simulink model "mm"  (R2023b)
settings: Solver=VariableStepAuto  StartTime=0.0  StopTime=10.0  RelTol=1e-3
undefined symbols (not defined in the file or in its folder): S, vsva2197, xcvc1902
libraries: aieBasic x3, vmcUtilities x1
settings Model: Creator=a.gnaneswaran  LastModifiedBy=a.gnaneswaran

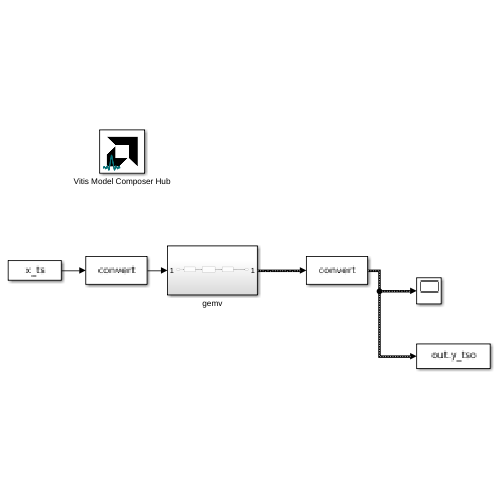
[thumbnail: Simulink's stored preview of the top-level diagram]
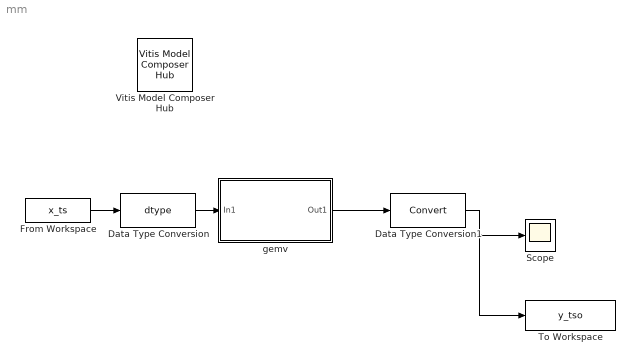
== system mm ==
  Data Type Conversion : DataTypeConversion  OutDataTypeStr=dtype  SaturateOnIntegerOverflow=off  RndMeth=Floor
  Data Type Conversion1 : DataTypeConversion  SaturateOnIntegerOverflow=off  RndMeth=Floor
  From Workspace : FromWorkspace  VariableName=x_ts  OutDataTypeStr=double  SampleTime=1
  Scope : Scope
  To Workspace : ToWorkspace  VariableName=y_tso  SaveFormat=Timeseries  SampleTime=1
      settings: Save2DSignal=2-D array (concatenate along first dimension)
  Vitis Model Composer Hub : vmcUtilities/Vitis Model Composer Hub  Tag=genX  CodeGeneration=off  SubsystemName=gemv  CompilationType=AIECompilation  ExportTypeV2=Graph Code  TargetDirectory=./code  exportDesign=off  analyzeDesign=on  validateDesignOnHw=off  ExportType=AI Engines  IpVendor=xilinx.com  IpLibrary=hls  IpVersion=1.0  IpHWLanguage=Verilog  AieCompilerOptions={}  AieSimulatorOptions={}  CreateTestbench=on  TestbenchStackSize=10  RunRtlSim=off  RunCSim=off  RunAieSim=on  AieSimTimeout=50000  RunAieSimProfiling=off  LaunchVitisAnalyzer=on  PlotOutput=off  RunX86Sim=off  X86SimTimeout=10  GenHwImage=off  GenLibadfXo=off  GenHwValidationCode=off  PlatformType=Not Specified  HwSystemType=Baremetal  HwValidationTarget=hw  ProjDevice=Versal VCK190 Evaluation Platform (xcvc1902-vsva2197-2MP-e-S)  ProjDevicePart=xcvc1902-vsva2197-2MP-e-S  AIEType=AIE  SamplePeriod=-1  ClockFrequency=200  DataPathParallelism=1  xilinxfamily=versalaicore  part=xcvc1902  speed=-2MP-e-S  package=vsva2197  directory=./netlist  testbench=off  incr_netlist=off  synthesis_tool=Vivado  clock_wrapper=Clock Enables  dbl_ovrd=According to Block Masks  dcm_input_clock_period=10  sysclk_period=10  simulink_period=1  eval_field=0  IPInfoJsonString="{\"AIESubsystem\":{\"SubsystemName\":\"gemv\",\"TargetDirectory\":\"./code\",\"SubsystemDir\":\"./code/ip/gemv\"},\"SubsystemTag\":\"AIENode\"}"  LogFileName=/home/a.gnaneswaran/aie_mc/mm/code/model_composer.log  NThreads=4
  gemv : Subsystem
  wires:
  From Workspace/1 -> Data Type Conversion/1
  Data Type Conversion1/1 -> To Workspace/1, Scope/1
  Data Type Conversion/1 -> gemv/1(In1)
  gemv/1(Out1) -> Data Type Conversion1/1

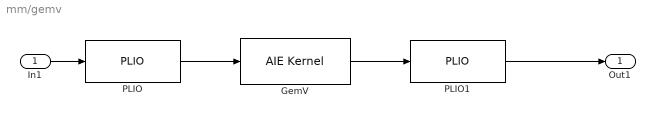
== system mm/gemv ==
  In1 : Inport
  GemV : aieBasic/AIE Kernel  KernelAllAttrs=|  PortNames={'in'; 'out'}  PortSerializedTypes={'{Q2{P{Tinput_stream{1{t{Bi8}}}}}}'; '{Q2{P{Toutput_stream{1{t{Bi8}}}}}}'}  PortWindowSizes={0.000000000000000000e+00, 0.000000000000000000e+00}  PortWindowMargins={0.000000000000000000e+00, 0.000000000000000000e+00}  PortSynchronicities={'auto', 'auto'}  PortSignalSizes={0.000000000000000000e+00; 1.280000000000000000e+02}  FunctionTemplateSpecKind=implicit  FunctionTemplateParamNames={'DX'; 'DY'}  FunctionTemplateParamKinds={'nontype'; 'nontype'}  FunctionTemplateParamTypes={'int'; 'int'}  FunctionTemplateParamValues={'128', '128'}  FunctionIndex=1  FunctionTabVisible=on  FunctionTemplateParamsVisible=on  FunctionDeclTypeOptions=|  FunctionDecl=|  FunctionTemplateParams={ 'DX', 'int', 'DX'; 'DY', 'int', 'DY' }  FunctionTemplateParamsEnables={'off', 'off', 'on';'off', 'off', 'on'}  PortAttrs={ 'input', 'in', 'input_stream_int8 * restrict', '', '', '', ''; 'output', 'out', 'output_stream_int8 * restrict', '', '', '', 'DY' }  PortAttrsEnables={'off', 'off', 'off', 'off', 'off', 'off', 'off';'off', 'off', 'off', 'off', 'off', 'off', 'on'}  SampleTime=-1  KernelHeaderFile=GemV.h  KernelFunction=GemV  KernelSourceFile=GemV.cpp  KernelSearchPaths={}  PreProcOptions={}  blockJsonConstraints="{\"type\":\"constraint\",\"constraintType\":\"stackSize\",\"sid\":\"16\",\"lhs\":{\"type\":\"stackSize\",\"args\":{\"type\":\"kernel\",\"name\":\"mm/gemv/GemV\",\"sid\":\"16\"}},\"rhs\":{\"type\":\"value\",\"args\":{\"type\":\"evaluable\",\"expr\":\"2048\",\"value\":2048}},\"equality\":true}"
      KernelAllAttrs=|
      | s[12;12;9;9;19;14;21;23;21;23;24;21;15;17;12;24;26;26;26;27;28;9;21;23;23;23;24;25;14;19;19;29]@FunctionNameDeclFileNamePortNamesPortTypesPortSerializedTypesPortDirectionsPortWindowSizeEnablesPortWindowMarginEnablesPortBufferSizeEnablesPortBufferMarginEnablesPortSynchronicityEnablesPortSignalSizeEnablesPortBufferSizesPortBufferMarginsFunctionDeclFunctionTemplateSpecKindFunctionTemplateParamNamesFunctionTemplateParamKindsFunctionTemplateParamTypesFunctionTemplateParamValuesFunctionTemplateParamEnablesClassDeclClassTemplateSpecKindClassTemplateParamNamesClassTemplateParamKindsClassTemplateParamTypesClassTemplateParamValuesClassTemplateParamEnablesClassCtorDeclsClassCtorParamNamesClassCtorParamTypesClassCtorParamSerializedTypes[1 1]@C[32 1]@t4@GemVt12@../../GemV.hC[2 1]@t2@int3@outC[2 1]@t28@input_stream_int8 * restrictt29@output_stream_int8 * restrictC[2 1]@t33@{Q2{P{Tinput_stream{1{t{Bi8}}}}}}t34@{Q2{P{Toutput_stream{1{t{Bi8}}}}}}C[2 1]@t5@inputt6@outputC[2 1]@l0@l0@C[2 1]@l0@l0@C[2 1]@l0@l0@C[2 1]@l0@l0@C[2 1]@l0@l0@C[2 1]@l0@l1@C[2 1]@nnC[2 1]@nnt106@template < int DX, int DY > 
      | void GemV(input_stream_int8 * restrict in, output_stream_int8 * restrict out)t8@implicitC[2 1]@t2@DXt2@DYC[2 1]@t7@nontypet7@nontypeC[2 1]@t3@intt3@intC[2 1]@nnC[2 1]@l1@l1@nne[0 1]@e[0 1]@e[0 1]@e[0 1]@e[0 1]@e[0 1]@e[0 1]@e[0 1]@e[0 1]@
      FunctionDeclTypeOptions=|
      | C[1 1]@t106@template < int DX, int DY > 
      | void GemV(input_stream_int8 * restrict in, output_stream_int8 * restrict out)
      FunctionDecl=|
      | template < int DX, int DY > 
      | void GemV(input_stream_int8 * restrict in, output_stream_int8 * restrict out)
  PLIO : aieBasic/PLIO  PlioWidth=32  PlioFreqSpec=on  PlioFreq=1000  ColLocation=0  channel=0  blockJsonConstraints=[]  deprecateConstraints=0
  PLIO1 : aieBasic/PLIO  PlioWidth=32  PlioFreqSpec=on  PlioFreq=1000  ColLocation=0  channel=0  blockJsonConstraints=[]  deprecateConstraints=0
  Out1 : Outport
  wires:
  In1/1 -> PLIO/1
  GemV/1 -> PLIO1/1
  PLIO/1 -> GemV/1
  PLIO1/1 -> Out1/1
